simulink model "FIGURA3_SUMATORIA"  (R2018a)
settings: Solver=VariableStepAuto  StartTime=0.0  StopTime=10.0  RelTol=1e-3
libraries: dspxfrm3 x1
settings Model: Creator=trigun  LastModifiedBy=trigun

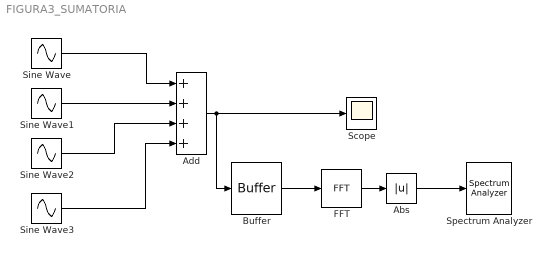
== system FIGURA3_SUMATORIA ==
  Abs : Abs
  Add : Sum  Inputs=++++
  Buffer : Buffer  OutputFrames=off
  FFT : dspxfrm3/FFT  FFTImplementation=Auto  CompMethod=Table lookup  TableOpt=NEW  TableOptActive=Speed  BitRevOrder=off  Normalize=off  InheritFFTLength=on  FFTLength=64  WrapInput=on  roundingMode=Floor  overflowMode=off  firstCoeffDataTypeStr=Inherit: Same word length as input  firstCoeffLastDataTypeStr=Inherit: Same word length as input  outputMin=[]  outputMax=[]
  Scope : Scope
  Sine Wave : Sin  Frequency=628.32  SampleTime=1/1000
  Sine Wave1 : Sin  Frequency=1884.96  SampleTime=1/1000
  Sine Wave2 : Sin  Frequency=3141.59  SampleTime=1/1000
  Sine Wave3 : Sin  Frequency=4398.23  SampleTime=1/1000
  Spectrum Analyzer : SpectrumAnalyzer
  wires:
  Sine Wave/1 -> Add/1
  Sine Wave1/1 -> Add/2
  Sine Wave2/1 -> Add/3
  Sine Wave3/1 -> Add/4
  Add/1 -> Buffer/1, Scope/1
  Buffer/1 -> FFT/1
  FFT/1 -> Abs/1
  Abs/1 -> Spectrum Analyzer/1
